simulink model "inverse_dynamics_with_observer"  (R2023b)
settings: Solver=VariableStepAuto  StartTime=0.0  StopTime=Tend_slk  RelTol=1e-3
undefined symbols (not defined in the file): A, B, C, D, Kpole, L, param, Ts_slk, x0, x_eq
settings Model: Creator=asus  LastModifiedBy=asus
settings OptimizationCC: ReuseModelBlockBuffer=off

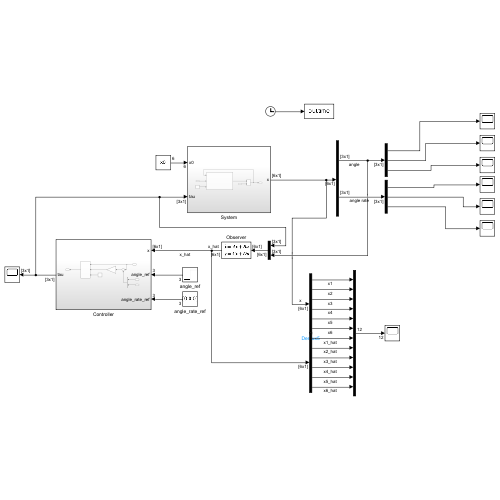
[thumbnail: Simulink's stored preview of the top-level diagram]
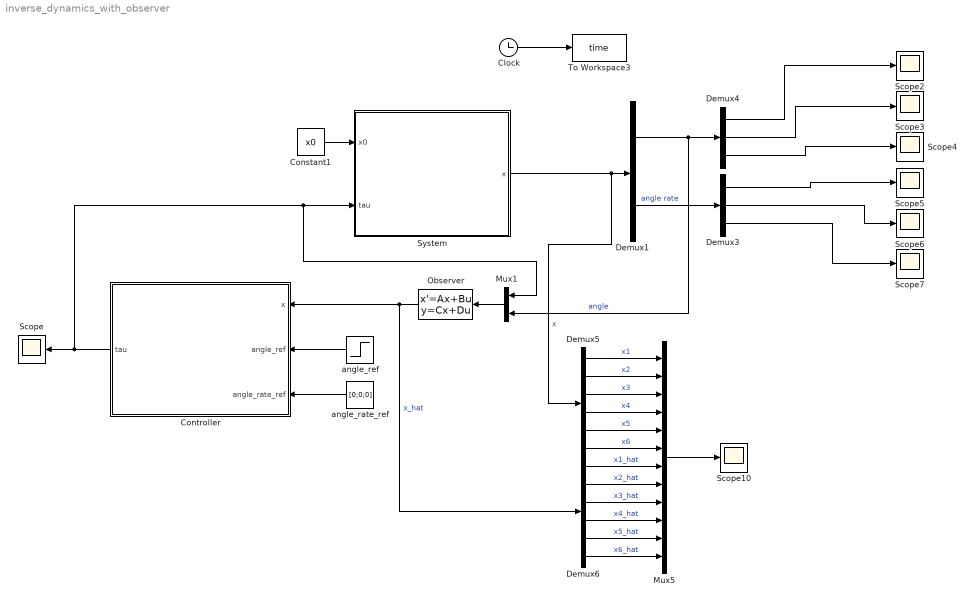
== system inverse_dynamics_with_observer ==
  Clock : Clock
  Constant1 : Constant  Value=x0
  Controller : Subsystem
  Demux1 : Demux  Outputs=2
  Demux3 : Demux  Outputs=3
  Demux4 : Demux  Outputs=3
  Demux5 : Demux  Outputs=6
  Demux6 : Demux  Outputs=6
  Mux1 : Mux  Inputs=2
  Mux5 : Mux  Inputs=12
  Observer : StateSpace  A=A-L*C  B=[B-L*D L]  C=eye(6)  D=zeros(6,6)  InitialCondition=0
  Scope{,2..7,10} (8 alike) : Scope
  System : Subsystem
  To Workspace3 : ToWorkspace  VariableName=time  SampleTime=Ts_slk
      settings: Save2DSignal=2-D array (concatenate along first dimension)
  angle_rate_ref : Constant  Value=[0;0;0]
  angle_ref : Step  Time=0  After=[1;1;1]*30*pi/180  SampleTime=0
  wires:
  Clock/1 -> To Workspace3/1
  Demux4/3 -> Scope4/1
  Demux4/1 -> Scope2/1
  Demux3/1 -> Scope5/1
  Demux3/3 -> Scope7/1
  Demux4/2 -> Scope3/1
  Demux3/2 -> Scope6/1
  Demux1/2 -> Demux3/1  "angle rate"
  Demux1/1 -> Mux1/2, Demux4/1  "angle"
  Controller/1(tau) -> Scope/1, Mux1/1, System/2("tau ")
  angle_ref/1 -> Controller/2(angle_ref)
  angle_rate_ref/1 -> Controller/3(angle_rate_ref)
  Constant1/1 -> System/1(x0)
  Mux1/1 -> Observer/1
  Demux6/6 -> Mux5/12  "x6_hat"
  Demux5/2 -> Mux5/2  "x2"
  Demux6/5 -> Mux5/11  "x5_hat"
  Demux5/1 -> Mux5/1  "x1"
  Demux5/4 -> Mux5/4  "x4"
  Demux5/6 -> Mux5/6  "x6"
  Demux6/3 -> Mux5/9  "x3_hat"
  Demux6/1 -> Mux5/7  "x1_hat"
  Observer/1 -> Controller/1(x), Demux6/1  "x_hat"
  Demux5/5 -> Mux5/5  "x5"
  Demux6/2 -> Mux5/8  "x2_hat"
  System/1(x) -> Demux5/1, Demux1/1  "x"
  Demux5/3 -> Mux5/3  "x3"
  Mux5/1 -> Scope10/1
  Demux6/4 -> Mux5/10  "x4_hat"

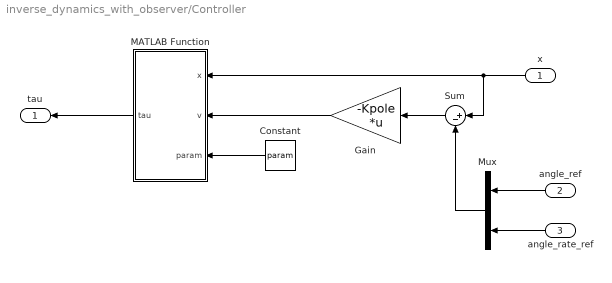
== system inverse_dynamics_with_observer/Controller ==
  x : Inport
  angle_ref : Inport  Port=2
  angle_rate_ref : Inport  Port=3
  Constant : Constant  Value=param
  Gain : Gain  Gain=-Kpole  Multiplication=Matrix(K*u) (u vector)
  MATLAB Function : MATLAB Function  TreatAsAtomicUnit=on
  Mux : Mux  Inputs=2
  Sum : Sum  Inputs=|+-
  tau : Outport
  wires:
  Constant/1 -> MATLAB Function/3(param)
  x/1 -> Sum/1, MATLAB Function/1(x)
  Gain/1 -> MATLAB Function/2(v)
  MATLAB Function/1(tau) -> tau/1
  Sum/1 -> Gain/1
  angle_ref/1 -> Mux/1
  Mux/1 -> Sum/2
  angle_rate_ref/1 -> Mux/2

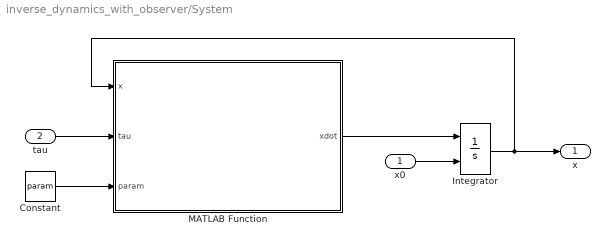
== system inverse_dynamics_with_observer/System ==
  x0 : Inport
  "tau " : Inport  Port=2
  Constant : Constant  Value=param
  Integrator : Integrator  InitialConditionSource=external  InitialCondition=x_eq
  MATLAB Function : MATLAB Function  TreatAsAtomicUnit=on
  x : Outport
  wires:
  Integrator/1 -> MATLAB Function/1(x), x/1
  MATLAB Function/1(xdot) -> Integrator/1
  "tau "/1 -> MATLAB Function/2(tau)
  Constant/1 -> MATLAB Function/3(param)
  x0/1 -> Integrator/2

== matlab function inverse_dynamics_with_observer/System/MATLAB Function ==
  data: x input; tau input; xdot output; param input
function xdot=quadcopter(x,tau,param)
% Inputs:
%           x       (model state)
%           tau     (torque)           
%           param   (model parameters)
%
% Outputs:  x_dot  (derivative of the state with respect to time)

% Parameters
g        =       9.81;           %  gravity acceleration (m/s^2)
Ixx      =       param(1,1);     %  moment of inertia 
Iyy      =       param(2,1);     %  moment of inertia
Izz      =       param(3,1);     %  moment of inertia 

% States
phi      =       x(1,1);     %  roll angle (rad)
theta    =       x(2,1);     %  pitch angle (rad)
psi      =       x(3,1);     %  yaw angle (rad)  
phi_dot  =       x(4,1);     %  roll rate (rad/s)
theta_dot=       x(5,1);     %  pitch rate (rad/s)
psi_dot  =       x(6,1);     %  yaw rate (rad/s)  

cph         =       cos(phi);
cth         =       cos(theta);
cps         =       cos(psi);
sph         =       sin(phi);
sth         =       sin(theta);
sps         =       sin(psi);  

% Coriolis matrix
C11=  0;
C12= (Iyy-Izz)*(theta_dot*cph*sph+psi_dot*sph^2*cth)+(Izz-Iyy)*psi_dot*cph^2*cth-Ixx*psi_dot*cth;
C13= (Izz-Iyy)*psi_dot*cph*sph*cth^2;
C21= (Izz-Iyy)*(theta_dot*cph*sph+psi_dot*sph*cth)+(Iyy-Izz)*psi_dot*cph^2*cth+Ixx*psi_dot*cth;
C22= (Izz-Iyy)*psi_dot*cph*sph;
C23= -Ixx*psi_dot*sth*cth+Iyy*psi_dot*sph^2*sth*cth+Izz*psi_dot*cph^2*sth*cth;
C31= (Iyy-Izz)*psi_dot*cth^2*sph*cph-Ixx*theta_dot*cth;
C32= (Izz-Iyy)*(theta_dot*cph*sph*sth+phi_dot*sph^2*cth)+(Iyy-Izz)*phi_dot*cph^2*cth+Ixx*psi_dot*sth*cth-Iyy*psi_dot*sph^2*sth*cth-Izz*psi_dot*cph^2*sth*cth;
C33= (Iyy-Izz)*phi_dot*cph*sph*cth^2-Iyy*theta_dot*sph^2*cth*sth-Izz*theta_dot*cph^2*cth*sth+Ixx*theta_dot*cth*sth;

C  = [C11 C12 C13;
    C21 C22 C23;
    C31 C32 C33];

% Inertia matrix
J11= Ixx;
J12= 0;
J13= -Ixx*sth;
J21= 0;
J22= Iyy*cph^2+Izz*sph^2;
J23= (Iyy-Izz)*cph*sph*cth;
J31= -Ixx*sth;
J32= (Iyy-Izz)*cph*sph*cth;
J33= Ixx*sth^2+Iyy*sph^2*cth^2+Izz*cph^2*cth^2;

J  = [J11 J12 J13;
    J21 J22 J23;
    J31 J32 J33];

%% Model Equations
invJ = [ (J22*J33 - J23*J32)/(J11*J22*J33 - J11*J23*J32 - J12*J21*J33 + J12*J23*J31 + J13*J21*J32 - J13*J22*J31), -(J12*J33 - J13*J32)/(J11*J22*J33 - J11*J23*J32 - J12*J21*J33 + J12*J23*J31 + J13*J21*J32 - J13*J22*J31),  (J12*J23 - J13*J22)/(J11*J22*J33 - J11*J23*J32 - J12*J21*J33 + J12*J23*J31 + J13*J21*J32 - J13*J22*J31);
         -(J21*J33 - J23*J31)/(J11*J22*J33 - J11*J23*J32 - J12*J21*J33 + J12*J23*J31 + J13*J21*J32 - J13*J22*J31),  (J11*J33 - J13*J31)/(J11*J22*J33 - J11*J23*J32 - J12*J21*J33 + J12*J23*J31 + J13*J21*J32 - J13*J22*J31), -(J11*J23 - J13*J21)/(J11*J22*J33 - J11*J23*J32 - J12*J21*J33 + J12*J23*J31 + J13*J21*J32 - J13*J22*J31);
         (J21*J32 - J22*J31)/(J11*J22*J33 - J11*J23*J32 - J12*J21*J33 + J12*J23*J31 + J13*J21*J32 - J13*J22*J31), -(J11*J32 - J12*J31)/(J11*J22*J33 - J11*J23*J32 - J12*J21*J33 + J12*J23*J31 + J13*J21*J32 - J13*J22*J31),  (J11*J22 - J12*J21)/(J11*J22*J33 - J11*J23*J32 - J12*J21*J33 + J12*J23*J31 + J13*J21*J32 - J13*J22*J31);];

xdot        = zeros(6,1);
xdot(1:3,1) = x(4:6,1);
xdot(4:6,1) = invJ*(tau - C*x(4:6,1));

== matlab function inverse_dynamics_with_observer/Controller/MATLAB Function ==
  data: x input; v input; tau output; param input
function tau = fcn(x,v,param)
% Import roll, pitch, yaw accelerations
% Parameters
g        =       9.81;           %  gravity acceleration (m/s^2)
Ixx      =       param(1,1);     %  moment of inertia 
Iyy      =       param(2,1);     %  moment of inertia
Izz      =       param(3,1);     %  moment of inertia 

% States
phi      =       x(1,1);     %  roll angle (rad)
theta    =       x(2,1);     %  pitch angle (rad)
psi      =       x(3,1);     %  yaw angle (rad)  
phi_dot  =       x(4,1);     %  roll rate (rad/s)
theta_dot=       x(5,1);     %  pitch rate (rad/s)
psi_dot  =       x(6,1);     %  yaw rate (rad/s)  

cph         =       cos(phi);
cth         =       cos(theta);
cps         =       cos(psi);
sph         =       sin(phi);
sth         =       sin(theta);
sps         =       sin(psi);

% Coriolis matrix
C11=  0;
C12= (Iyy-Izz)*(theta_dot*cph*sph+psi_dot*sph^2*cth)+(Izz-Iyy)*psi_dot*cph^2*cth-Ixx*psi_dot*cth;
C13= (Izz-Iyy)*psi_dot*cph*sph*cth^2;
C21= (Izz-Iyy)*(theta_dot*cph*sph+psi_dot*sph*cth)+(Iyy-Izz)*psi_dot*cph^2*cth+Ixx*psi_dot*cth;
C22= (Izz-Iyy)*psi_dot*cph*sph;
C23= -Ixx*psi_dot*sth*cth+Iyy*psi_dot*sph^2*sth*cth+Izz*psi_dot*cph^2*sth*cth;
C31= (Iyy-Izz)*psi_dot*cth^2*sph*cph-Ixx*theta_dot*cth;
C32= (Izz-Iyy)*(theta_dot*cph*sph*sth+phi_dot*sph^2*cth)+(Iyy-Izz)*phi_dot*cph^2*cth+Ixx*psi_dot*sth*cth-Iyy*psi_dot*sph^2*sth*cth-Izz*psi_dot*cph^2*sth*cth;
C33= (Iyy-Izz)*phi_dot*cph*sph*cth^2-Iyy*theta_dot*sph^2*cth*sth-Izz*theta_dot*cph^2*cth*sth+Ixx*theta_dot*cth*sth;

C  = [C11 C12 C13;
    C21 C22 C23;
    C31 C32 C33];

% Inertia matrix
J11= Ixx;
J12= 0;
J13= -Ixx*sth;
J21= 0;
J22= Iyy*cph^2+Izz*sph^2;
J23= (Iyy-Izz)*cph*sph*cth;
J31= -Ixx*sth;
J32= (Iyy-Izz)*cph*sph*cth;
J33= Ixx*sth^2+Iyy*sph^2*cth^2+Izz*cph^2*cth^2;

J  = [J11 J12 J13;
    J21 J22 J23;
    J31 J32 J33];

% control law
tau = zeros(3,1);
tau = J*v+C*x(4:6,1);
